simulink model "simulation"  (R2025b)
settings: Solver=VariableStepAuto  StartTime=0.0  StopTime=50  RelTol=1e-3
values from neighbouring files (symbols this model uses):
  A_1 = [zeros(2) eye(2) ... (first row only)    [model.m]
  Ad = s2.A    [model.m]
  B_1 = [0;0 ... (first row only)    [model.m]
  Bd = s2.B    [model.m]
  Cd = s2.C    [model.m]
  Dd = s2.D    [model.m]
  gamma = 0.999    [model.m]
  K_corr = acker(Ad,Bd,poles_souhaites)    [model.m]
  K_PWM = 8.087    [model.m]
  Psi0 = deg2rad(8)    [model.m]
  s1 = ss(A_1, B_1, eye(4), zeros(4,1))    [model.m]
  S_corr = inv([1 0 0 0]*inv(eye(4)-Ad+Bd*K_corr)*Bd)    [model.m]
  Ts = 0.004    [model.m]
undefined symbols (not defined in the file or in its folder): DiscIntNeverNeededParam
libraries: simulink x1
settings Model: Creator=loic  LastModifiedBy=carol
settings SolverCC: AlgebraicLoopSolver=TrustRegion
settings DataIOCC: ReturnWorkspaceOutputs=off
settings DebuggingCC: UnconnectedInputMsg=warning  UnconnectedOutputMsg=warning  UnconnectedLineMsg=warning  ArithmeticOperatorsInVariantConditions=warning
settings ModelReferenceCC: EnableRefExpFcnMdlSchedulingChecks=on
settings SFSimCC: SimUseLocalCustomCode=off  CustomCodeUndefinedFunction=UseInterfaceOnly
settings RTWCC: RTWUseLocalCustomCode=off  GPUComputeCapability=3.5
settings CodeAppCC: StateflowObjectComments=on

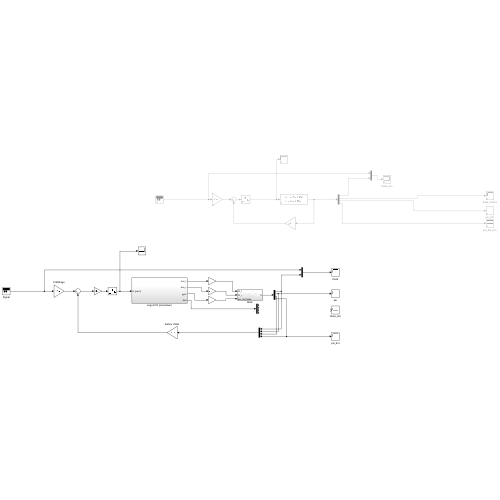
[thumbnail: Simulink's stored preview of the top-level diagram]
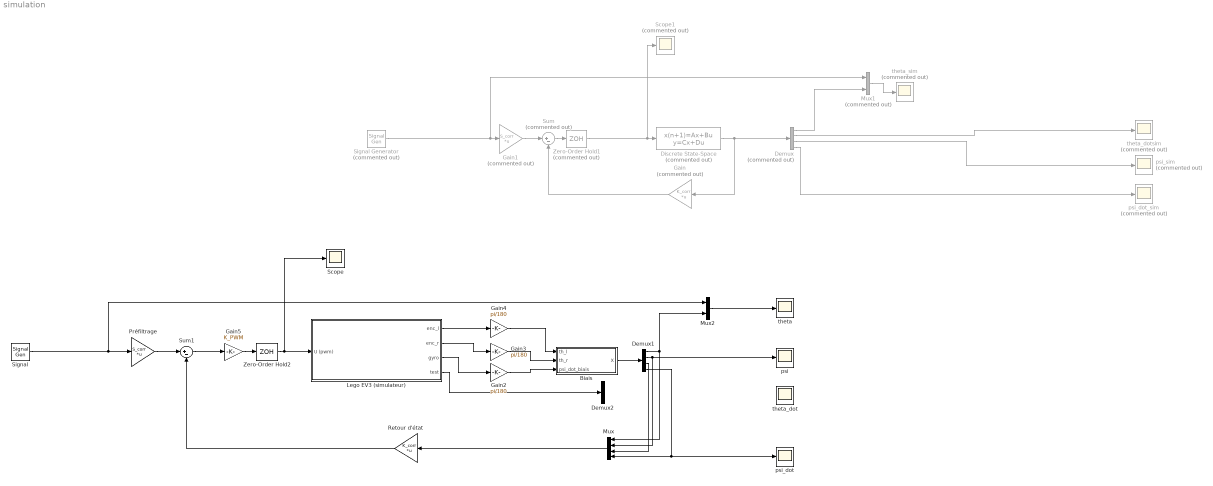
== system simulation ==
  Biais : Subsystem
  Demux : Demux  Commented=on
  Demux1 : Demux
  Demux2 : Demux
  Discrete State-Space : DiscreteStateSpace  Commented=on  A=Ad  B=Bd  C=Cd  D=Dd  InitialCondition=[0 Psi0 0 0]  SampleTime=Ts
  Gain : Gain  Commented=on  Gain=K_corr  Multiplication=Matrix(K*u)
  Gain1 : Gain  Commented=on  Gain=S_corr  Multiplication=Matrix(K*u)
  Gain2 : Gain  Gain=pi/180
  Gain3 : Gain  Gain=pi/180
  Gain4 : Gain  Gain=pi/180
  Gain5 : Gain  Gain=K_PWM
  Lego EV3 (simulateur) : Subsystem
  Mux : Mux
  Mux1 : Mux  Commented=on  Inputs=2
  Mux2 : Mux  Inputs=2
  Préfiltrage : Gain  Gain=S_corr  Multiplication=Matrix(K*u)
  Retour d'état : Gain  Gain=K_corr  Multiplication=Matrix(K*u)
  Scope : Scope
      settings: ActiveDisplayYMinimum=-623.65580691886532  ActiveDisplayYMaximum=405.37809192653361  DataLoggingVariableName=ScopeData11
  Scope1 : Scope  Commented=on
      settings: ActiveDisplayYMinimum=-125  ActiveDisplayYMaximum=125  DataLoggingVariableName=ScopeData3
  Signal : SignalGenerator  WaveForm=square  Frequency=0.1
  Signal Generator : SignalGenerator  Commented=on  WaveForm=square  Frequency=0.1
  Sum : Sum  Commented=on  Inputs=|+-
  Sum1 : Sum  Inputs=|+-
  Zero-Order Hold1 : ZeroOrderHold  Commented=on  SampleTime=Ts
  Zero-Order Hold2 : ZeroOrderHold  SampleTime=Ts
  psi : Scope
      settings: DataLoggingVariableName=ScopeData5
  psi_dot : Scope
      settings: ActiveDisplayYMinimum=-4.9328102341799545  ActiveDisplayYMaximum=4.93528931485691  DataLoggingVariableName=ScopeData7
  psi_dot_sim : Scope  Commented=on
      settings: ActiveDisplayYMinimum=-6.3751867241571265  ActiveDisplayYMaximum=3.4383633274939918  DataLoggingVariableName=ScopeData9
  psi_sim : Scope  Commented=on
      settings: ActiveDisplayYMinimum=-37.776698851768359  ActiveDisplayYMaximum=26.864683122273959  DataLoggingVariableName=ScopeData8
  theta : Scope
      settings: ActiveDisplayYMinimum=-4.5668612020924009  ActiveDisplayYMaximum=1.4843755837362789  DataLoggingVariableName=ScopeData4
  theta_dot : Scope
      settings: DataLoggingVariableName=ScopeData6
  theta_dotsim : Scope  Commented=on
      settings: ActiveDisplayYMinimum=-0.15525930149524045  ActiveDisplayYMaximum=0.17239141145452266  DataLoggingVariableName=ScopeData10
  theta_sim : Scope  Commented=on
      settings: ActiveDisplayYMinimum=-1.9770833765148397  ActiveDisplayYMaximum=1.7165552329578189
  wires:
  Signal Generator/1 -> Mux1/1, Gain1/1
  Sum/1 -> Zero-Order Hold1/1
  Gain/1 -> Sum/2
  Mux1/1 -> theta_sim/1
  Gain1/1 -> Sum/1
  Discrete State-Space/1 -> Demux/1, Gain/1
  Zero-Order Hold1/1 -> Scope1/1, Discrete State-Space/1
  Demux/1 -> Mux1/2
  Lego EV3 (simulateur)/1(enc_l) -> Gain4/1
  Lego EV3 (simulateur)/2(enc_r) -> Gain3/1
  Lego EV3 (simulateur)/3(gyro) -> Gain2/1
  Gain4/1 -> Biais/1(th_l)
  Gain3/1 -> Biais/2(th_r)
  Gain2/1 -> Biais/3(psi_dot_biais)
  Préfiltrage/1 -> Sum1/1
  Signal/1 -> Mux2/1, Préfiltrage/1
  Mux2/1 -> theta/1
  Retour d'état/1 -> Sum1/2
  Sum1/1 -> Gain5/1
  Gain5/1 -> Zero-Order Hold2/1
  Demux/4 -> psi_dot_sim/1
  Demux/2 -> theta_dotsim/1
  Demux/3 -> psi_sim/1
  Zero-Order Hold2/1 -> Lego EV3 (simulateur)/1(U (pwm)), Scope/1
  Biais/1(X) -> Demux1/1
  Lego EV3 (simulateur)/4(test) -> Demux2/1
  Mux/1 -> Retour d'état/1
  Demux1/1 -> Mux2/2, Mux/1
  Demux1/4 -> Mux/4, psi_dot/1
  Demux1/2 -> psi/1, Mux/2
  Demux1/3 -> Mux/3

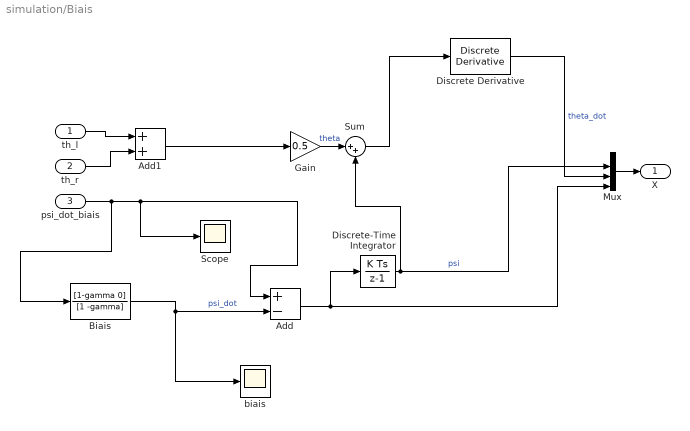
== system simulation/Biais ==
  th_l : Inport
  th_r : Inport  Port=2
  psi_dot_biais : Inport  Port=3
  Add : Sum  Inputs=+-
  Add1 : Sum
  Biais : DiscreteTransferFcn  Numerator=[1-gamma 0]  Denominator=[1 -gamma]
  Discrete Derivative : simulink/Quick Insert/Discrete/Discrete Derivative  gainval=1.0  ICPrevScaledInput=0.0  OutMin=[]  OutMax=[]  OutDataType=fixdt(1, 16)  OutScaling=2^-10  DoSatur=off
  Discrete-Time Integrator : DiscreteIntegrator  SampleTime=Ts  ICPrevOutput=DiscIntNeverNeededParam  ICPrevScaledInput=DiscIntNeverNeededParam
  Gain : Gain  Gain=0.5
  Mux : Mux
  Scope : Scope
      settings: ActiveDisplayYMinimum=-1  ActiveDisplayYMaximum=1  DataLoggingVariableName=ScopeData13
  Sum : Sum  Inputs=|++
  biais : Scope
      settings: ActiveDisplayYMinimum=-0.1164059395354744  ActiveDisplayYMaximum=0.0646369691442869  DataLoggingVariableName=ScopeData12
  X : Outport
  wires:
  th_l/1 -> Add1/1
  th_r/1 -> Add1/2
  Add1/1 -> Gain/1
  Mux/1 -> X/1
  Discrete Derivative/1 -> Mux/3  "theta_dot"
  Discrete-Time Integrator/1 -> Sum/2, Mux/2  "psi"
  psi_dot_biais/1 -> Biais/1, Scope/1, Add/1
  Biais/1 -> Add/2, biais/1  "psi_dot"
  Add/1 -> Mux/4, Discrete-Time Integrator/1
  Gain/1 -> Sum/1  "theta"
  Sum/1 -> Discrete Derivative/1

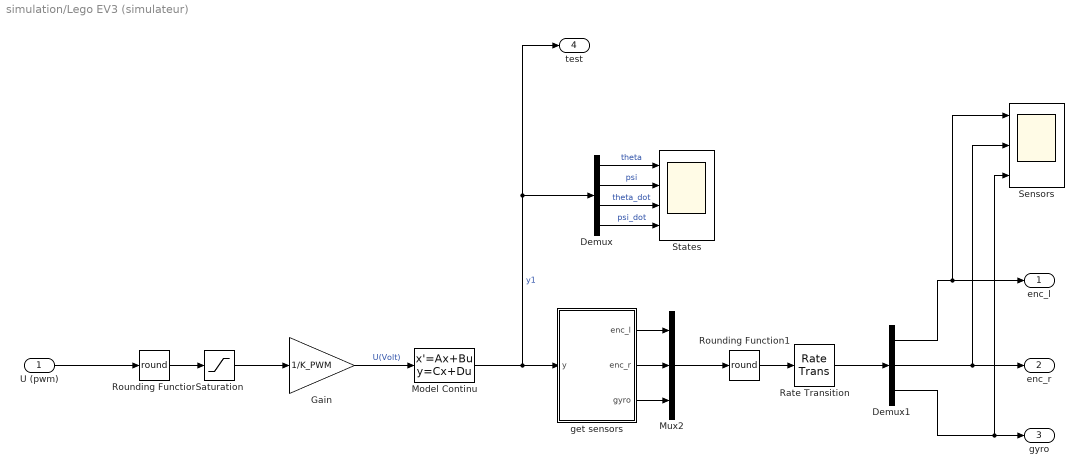
== system simulation/Lego EV3 (simulateur) ==
  U (pwm) : Inport
  Demux : Demux
  Demux1 : Demux  Outputs=3
  Gain : Gain  Gain=1/K_PWM
  Model Continu : StateSpace  A=A_1  B=B_1  C=eye(4)  D=s1.D  InitialCondition=[0 Psi0 0 0]
  Mux2 : Mux  Inputs=3
  Rate Transition : RateTransition  OutPortSampleTime=Ts
  Rounding Function : Rounding  Operator=round
  Rounding Function1 : Rounding  Operator=round
  Saturation : Saturate  UpperLimit=100  LowerLimit=-100
  Sensors : Scope  NumInputPorts=3
      settings: ActiveDisplayYMinimum=-115  ActiveDisplayYMaximum=265
  States : Scope  NumInputPorts=4
      settings: ActiveDisplayYMinimum=-18.762173178074935  ActiveDisplayYMaximum=8.1937673053565856  DataLoggingVariableName=ScopeData2
  get sensors : MATLAB Function  TreatAsAtomicUnit=on
  enc_l : Outport
  enc_r : Outport  Port=2
  gyro : Outport  Port=3
  test : Outport  Port=4
  wires:
  Model Continu/1 -> test/1, Demux/1, get sensors/1(y)  "y1"
  Gain/1 -> Model Continu/1  "U(Volt)"
  Saturation/1 -> Gain/1
  U (pwm)/1 -> Rounding Function/1
  get sensors/3(gyro) -> Mux2/3
  Demux/4 -> States/4  "psi_dot"
  Rounding Function1/1 -> Rate Transition/1
  Demux/2 -> States/2  "psi"
  Demux/3 -> States/3  "theta_dot"
  Demux/1 -> States/1  "theta"
  get sensors/1(enc_l) -> Mux2/1
  get sensors/2(enc_r) -> Mux2/2
  Rounding Function/1 -> Saturation/1
  Mux2/1 -> Rounding Function1/1
  Rate Transition/1 -> Demux1/1
  Demux1/1 -> Sensors/1, enc_l/1
  Demux1/2 -> Sensors/2, enc_r/1
  Demux1/3 -> Sensors/3, gyro/1

== matlab function simulation/Lego EV3 (simulateur)/get sensors ==
  data: enc_l output; enc_r output; y input; gyro output; R parameter
function [enc_l, enc_r, gyro] = sensors(y, R)
enc_l = rad2deg(y(1) - y(2));
enc_r = rad2deg(y(1) - y(2));
gyro  = rad2deg(y(4));
